simulink model "tankModelSimulink"  (R2021a)
settings: Solver=VariableStepAuto  StartTime=0.0  StopTime=10  RelTol=1e-3
values from neighbouring files (symbols this model uses):
  A = [1 1 ... (first row only)    [LQR2x2.m]    (also in LQR3x3.m = [-0.1 0 0; PID.m = [-0.1 -0.12; tankModel.m = 5)
  c = -a*(2*g)^0.5/A    (= -0.885889383614)    [tankModel.m]
  d = a*(2*g)^0.5    (= 4.42944691807)    [tankModel.m]
settings Model: Creator=lukar  LastModifiedBy=lukar

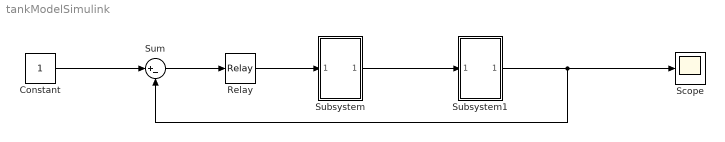
== system tankModelSimulink ==
  Constant : Constant
  Relay : Relay
  Scope : Scope
  Subsystem : Subsystem
  Subsystem1 : Subsystem
  Sum : Sum  Inputs=|+-
  wires:
  Subsystem/1(Out1) -> Subsystem1/1(In1)
  Subsystem1/1(Out1) -> Scope/1, Sum/2
  Relay/1 -> Subsystem/1(In1)
  Sum/1 -> Relay/1
  Constant/1 -> Sum/1

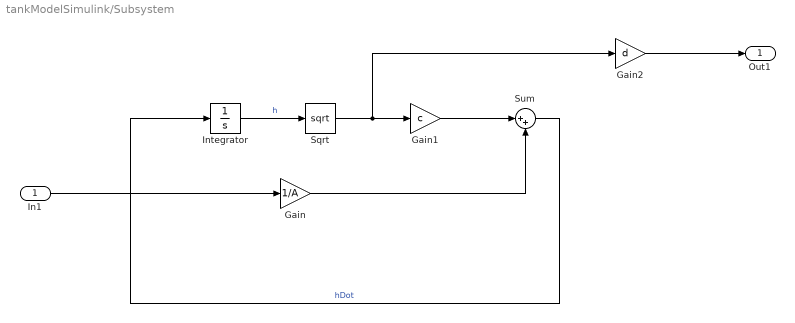
== system tankModelSimulink/Subsystem ==
  In1 : Inport
  Gain : Gain  Gain=1/A
  Gain1 : Gain  Gain=c
  Gain2 : Gain  Gain=d
  Integrator : Integrator  InitialCondition=3
  Sqrt : Sqrt  SaturateOnIntegerOverflow=on
  Sum : Sum  Inputs=|++
  Out1 : Outport
  wires:
  Gain1/1 -> Sum/1
  Sqrt/1 -> Gain2/1, Gain1/1
  Sum/1 -> Integrator/1  "hDot"
  Integrator/1 -> Sqrt/1  "h"
  Gain/1 -> Sum/2
  In1/1 -> Gain/1
  Gain2/1 -> Out1/1

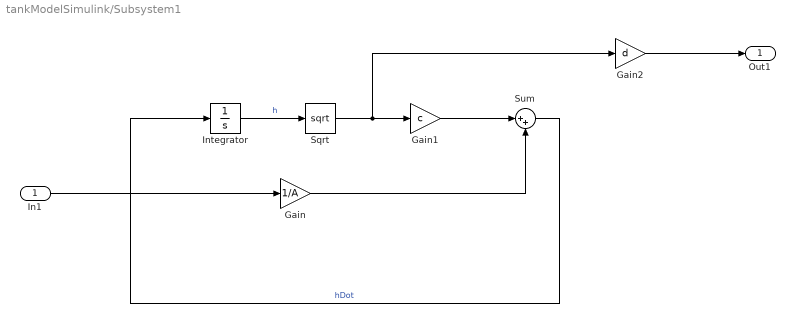
== system tankModelSimulink/Subsystem1 ==
  In1 : Inport
  Gain : Gain  Gain=1/A
  Gain1 : Gain  Gain=c
  Gain2 : Gain  Gain=d
  Integrator : Integrator  InitialCondition=3
  Sqrt : Sqrt  SaturateOnIntegerOverflow=on
  Sum : Sum  Inputs=|++
  Out1 : Outport
  wires:
  Gain1/1 -> Sum/1
  Sqrt/1 -> Gain2/1, Gain1/1
  Sum/1 -> Integrator/1  "hDot"
  Integrator/1 -> Sqrt/1  "h"
  Gain/1 -> Sum/2
  In1/1 -> Gain/1
  Gain2/1 -> Out1/1
